simulink library "SUB_ECU_L4_MABX_HW_Interface_PIC_PB"  (R2018a)
settings: Solver=VariableStepAuto  StartTime=0.0  StopTime=10.0  RelTol=1e-3
PostLoadFcn:
  | , if any(exist('dsrtsu_mdlpostloadfcn', 'file') == [2, 3, 6]), try dsrtsu_mdlpostloadfcn('Execute', bdroot); catch fprintf('Error in PostLoadFcn (dsrtsu_mdlpostloadfcn) for model "%s":\n %s\n', bdroot, lasterr); end, end,
undefined symbols (not defined in the file or in its folder): CANR_PROPB_REAX_3_13_CHANNEL_APV, CANR_PROPB_REAX_4_13_CHANNEL_APV, CANR_PROPB_XPR_1_50_CHANNEL_APV, ENUM_CAN_RX_T, ENUM_CAN_TX_T, ENUM_REAX_OPERATION_MODE_T, ENUM_SIGNAL_HEALTH_T, ENUM_XBR_CONTROL_MODE_T, ENUM_XBR_EBI_MODE_T, ENUM_XBR_PASS_THROUGH_ACTIVE_T, ENUM_XBR_PRIORITY_T, ENUM_XPR_INHIBIT_PARK_MANUAL_T, ENUM_XPR_INHIBIT_UNPARK_MANUAL_T, ENUM_XPR_PARK_MANUAL_T, ENUM_XPR_UNPARK_MANUAL_T, PROPB_REAX_1_E4_DES_POS_SIG_SRC_APV, PROPB_REAX_1_E4_DESIRED_OPMODE_APV, PROPB_REAX_1_E4_DESIRED_POSITION_APV, PROPB_REAX_CHANNEL_APV, ptc_matlab_lib
libraries: PTC_MBDS_LIB x293, rtican x158, simulink x61, EmE_MBD_Blockset x38, rti1401lib_dio_type4 x14, simulink_need_slupdate x7, $bdroot x5, rti1401lib_adc_type4 x3, rtmapslib x3, dsa_tcpip_lib x2, SUB_ECU_L4_MABX_HW_Interface_PTC_1571 x1, rtitasklib x1
(part 29 of 49)

== system SUB_ECU_L4_MABX_HW_Interface_PIC_PB/INPUTS_PIC_PB/CAN_PIC_PB/CAN_RX_AIR1_31/RX_CAN_1 ==
  Enable : Inport
  AIR1 : rtican/RTICAN Receive (RX)   Reserved1=[]  Reserved2=[]  Reserved3=[]  Reserved4=[]  SfcnMessage=[]  Msg_Struct=[]  BoardTypeNo=[]  BoardNo=[]  ChannelNo=[]  Parameters=[]  DialogFcn=[]  UnitName=[]  Revision=[]  UnitValues=[]  DSProperties=struct('RTI',struct('Version',uint32(5),'BlockType',struct('isSLSource',uint8(1),'isSLSink',uint8(1),'isHWSource',uint8(0),'isHWSink',uint8(0),'isSetup',uint8(0),'isInline',uint8(1),'isNonInline',uint8(0),'isInterrupt',uint8(0),'isChannelwise',uint8(0)),'IOBoardType','RTICAN','UnitType','MESSAGE','Identifier','RX','DialogType','MSVC','BlockSet','RTICAN','SlaveProcessor','CAN'))  RTIBlockInterface=struct('OutputPortsWidth',int32([1 1 1 1 1 1 1 1 1 1 1]),'OutputPortsActive',ones(1,11),'OutputPortsName',{{'PneumaticSupplyPress','ParkingAnd_orTrailerAirPress','ServiceBrakeCircuit1AirPress','ServiceBrakeCircuit2AirPress','AuxEquipmentSupplyPress','AirSuspensionSupplyPress','AirCompressorStatus','PowertrainCircuitAirSupplyPress',['RX status'],['RX time'],['RX delta time']}},'OutputPortsDataType',{{'SS_DOUBLE','SS_DOUBLE','SS_DOUBLE','SS_DOUBLE','SS_DOUBLE','SS_DOUBLE','SS_DOUBLE','SS_DOUBLE','SS_DOUBLE','SS_DOUBLE','SS_DOUBLE'}},'OutputPortsLabel',{{'PneumaticSupplyPress','ParkingAnd_orTrailerAirPress','ServiceBrakeCircuit1AirPress','ServiceBrakeCircuit2AirPress','AuxEquipmentSupplyPress','AirSuspensionSupplyPress','AirCompressorStatus','PowertrainCircuitAirSupplyPress','','',''}},'OutputPortsLabelMode','ON','InputPortsWidth',int32(0),'InputPortsActive',0,'DialogFcn','rtican_message_interface_gui','BlockDisplay',{{'','center'}},'IconTransparency','on','ParameterTunableNames',{{}},'InitLevel',3,'BlockName',struct('Token',{{'AIR1'}}),'SampleTime',{{-1}},'TriggerPort',{{'none'}},'EnablePort',{{'yes'}})  RTIBlockParameters="struct('BoardTypeNo',{{1,'OFF',[]}},'BoardNo',{{1,'ON',[1 16]}},'ChannelNo',{{1,'ON',[1 2]}},'Parameters',{{struct('DataFileSupport',struct('DataFileSelectedMaster',1,'DataFileSelectedLocal',0,'DataFileName',['c:\\data\\truck1571\\dbc\\mabx_can1.dbc|c:\\data\\svn\\powertrainsys\\trunk\\src\\projects_rcp\\my2017_rcp\\dbc files\\j1939.dbc|'],'DataFileDate',{{{['24-Jan-2018 14:59:01']},{['24-Aug-2017 12:01:59']}}},'SelectedFile',['..\\svn\\powertrainsys\\trunk\\src\\projects_rcp\\my2017_rcp\\dbc files\\j1939.dbc']),'Options',struct('StatusSelected',1,'TimeSelected',1,'DeltaTimeSelected',1,'BytePortSelected',0,'MessageLengthSelected',0,'TriggerPort',struct('Selected',0,'TriggerType',0),'UserCoding',struct('Selected',0,'InterfaceFile','UserDecodingFile','FcnName','UserDecodeFcn','InportSelected',0,'InportWidth',1,'OutportSelected',0,'OutportWidth',1),'EnablePortSelected',1,'SignalOnPortnameSelected',1,'UseRXService',1),'Message',struct('MsgOnBlocknameSelected',1,'MsgName','AIR1','MsgIdFormat',1,'MsgId',419343921,'MsgLength',8,'NumSignals',8,'SampleTime',-1,'Signal',struct('SgnName',{'PneumaticSupplyPress','ParkingAnd_orTrailerAirPress','ServiceBrakeCircuit1AirPress','ServiceBrakeCircuit2AirPress','AuxEquipmentSupplyPress','AirSuspensionSupplyPress','AirCompressorStatus','PowertrainCircuitAirSupplyPress'},'SgnStartBit',{0,8,16,24,32,40,48,56},'SgnLength',{8,8,8,8,8,8,2,8},'SgnType',{0,0,0,0,0,0,0,0},'ModeValue',{-1,-1,-1,-1,-1,-1,-1,-1},'DataType',{0,0,0,0,0,0,0,0},'ByteLayout',{0,0,0,0,0,0,0,0},'Factor',{8,8,8,8,8,8,1,8},'Offset',{0,0,0,0,0,0,0,0},'SgnComment',{{['The pneumatic pressure in the main reservoir, sometimes referred to as the wet tank.']},{['The pneumatic pressure in the circuit or reservoir for the parking brake and/or the trailer supply.']},{['The pneumatic pressure in the primary service brake circuit or reservoir, supplying the rear axle.']},{['The pneumatic pressure in the secondary service brake circuit or reservoir, supplying the front axle.']},{['The pneumatic pressure in the auxiliary circuit.']},{['The pneumatic pressure in the circuit for the electronically controlled air suspension system.']},{['Indicates whether the air compressor is actively compressing air.  ' char(10) '' char(10) '00     Compressor not active' char(10) '01     Compressor active' char(10) '10     Error indicator' char(10) '11     Not available']},{['Supply pressure to carry the pressure information for the powertrain circuit. This circuit typically would feed powertrain components such as throttles, gearbox actuators and aftertreatment actuators for EGR and SCR systems.']}},'SgnUnit',{'kPa','kPa','kPa','kPa','kPa','kPa','','kPa'},'Min',{0,0,0,0,0,0,0,0},'Max',{2000,2000,2000,2000,2000,2000,3,2000},'SLDataType',{'SS_DOUBLE','SS_DOUBLE','SS_DOUBLE','SS_DOUBLE','SS_DOUBLE','SS_DOUBLE','SS_DOUBLE','SS_DOUBLE'}),'MsgIdNumFormat',1,'MsgComment',{{['Air Supply Pressure' char(10) 'Air Supply Pressure']}}),'Version',1.2,'general',struct('isFromLib',0)),'OFF',[]}},'GroupId',{{struct('Group',{{'RTICAN'}},'No',1,'Behavior',{{'NAMECHANGE'}},'BlockType',{{'SINK'}},'NameChangeFlag',0),'OFF',[]}},'SFcnRTICANMessage',{{struct('MsgType','RX','SFcnPortType','Scalar','MsgName','AIR1','MsgIdFormat','XTD','MsgId',419343921,'MsgLength',8,'NumSignals',8,'SampleTime',-1,'Signal',struct('SgnName',{'PneumaticSupplyPress','ParkingAnd_orTrailerAirPress','ServiceBrakeCircuit1AirPress','ServiceBrakeCircuit2AirPress','AuxEquipmentSupplyPress','AirSuspensionSupplyPress','AirCompressorStatus','PowertrainCircuitAirSupplyPress'},'SgnStartBit',{0,8,16,24,32,40,48,56},'SgnLength',{8,8,8,8,8,8,2,8},'SgnType',{'standard','standard','standard','standard','standard','standard','standard','standard'},'ModeValue',{-1,-1,-1,-1,-1,-1,-1,-1},'DataType',{['unsigned int'],['unsigned int'],['unsigned int'],['unsigned int'],['unsigned int'],['unsigned int'],['unsigned int'],['unsigned int']},'ByteLayout',{['little endian'],['little endian'],['little endian'],['little endian'],['little endian'],['little endian'],['little endian'],['little endian']},'Factor',{8,8,8,8,8,8,1,8},'Offset',{0,0,0,0,0,0,0,0},'SLDataType',{'SS_DOUBLE','SS_DOUBLE','SS_DOUBLE','SS_DOUBLE','SS_DOUBLE','SS_DOUBLE','SS_DOUBLE','SS_DOUBLE'}),'StatusSelected','yes','TimeSelected','yes','DeltaTimeSelected','yes','BytePortSelected','no','MessageLengthSelected','no','TriggerPort',struct('Selected','no','TriggerType',0),'UserCoding',struct('Selected','no','InterfaceFile','UserDecodingFile','FcnName','UserDecodeFcn','InportSelected','no','InportWidth',1,'OutportSelected','no','OutportWidth',1),'EnablePortSelected','yes','UseRXService','yes','BoardType','DS1','BoardNo',1,'ControllerNo',1),'OFF',[]}},'TLCFileName',{{'rtican_rx_message','OFF',[]}})"  RTISFcnParameters=struct('SFcnRTICANMessage','struct','TLCFileName','char')  RTIBlockParaDefault=struct('BoardTypeNo',4302,'BoardNo',1,'ChannelNo',1,'Parameters',struct('DataFileSupport',struct('DataFileSelectedMaster',0,'DataFileSelectedLocal',0,'DataFileName','','DataFileDate','','SelectedFile',['<no file selected>']),'Options',struct('StatusSelected',1,'TimeSelected',1,'DeltaTimeSelected',1,'BytePortSelected',0,'MessageLengthSelected',0,'TriggerPort',struct('Selected',0,'TriggerType','rising'),'UserCoding',struct('Selected',0,'InterfaceFile','UserDecodingFile','FcnName','UserDecodeFcn','InportSelected',0,'InportWidth',1,'OutportSelected',0,'OutportWidth',1),'EnablePortSelected',0,'SignalOnPortnameSelected',1,'UseRXService',0),'Message',struct('MsgOnBlocknameSelected',0,'MsgName',['RX Message'],'MsgIdFormat',0,'MsgId',100,'MsgLength',8,'NumSignals',1,'SampleTime',-1,'Signal',struct('SgnName',['RX signal'],'SgnStartBit',0,'SgnLength',8,'SgnType',0,'ModeValue',-1,'DataType',0,'SLDataType','SS_DOUBLE','ByteLayout',0,'Factor',1,'Offset',0,'Min',0,'Max',255,'SgnComment',{{}},'SgnUnit',''),'MsgIdNumFormat',0,'MsgComment',{{''}}),'Version',1.2,'general',struct('isFromLib',1)),'GroupId',struct('Group',{{'RTICAN'}},'No',1,'Behavior',{{'NAMECHANGE'}},'BlockType',{{'SINK'}},'NameChangeFlag',0),'SFcnRTICANMessage',struct('MsgType','RX','MsgName',['RX Message'],'MsgIdFormat','STD','MsgId',100,'MsgLength',8,'NumSignals',1,'SampleTime',-1,'Signal',struct('SgnName',['RX signal'],'SgnStartBit',0,'SgnLength',8,'SgnType','standard','ModeValue',-1,'DataType',['unsigned int'],'ByteLayout',['little endian'],'SLDataType','SS_DOUBLE','Factor',1,'Offset',0),'StatusSelected','yes','TimeSelected','yes','DeltaTimeSelected','yes','BytePortSelected','no','MessageLengthSelected','no','EnablePortSelected','no','UserCoding',struct('Selected','no','InterfaceFile','UserDecodingFile','FcnName','UserDecodeFcn','InportSelected','no','InportWidth',1,'OutportSelected','no','OutportWidth',1),'TriggerPort',struct('Selected','no','TriggerType','rising'),'UseRXService','no','BoardType','DS4302','BoardNo',1,'ControllerNo',1,'SFcnPortType','Scalar'),'TLCFileName','rtican_rx_message')
      settings: AttributesFormatString=Group Id: RTICAN1\n  SourceProductName=dSPACE RTI CAN Blockset
  Bus Creator : BusCreator  Inputs=8
  Bus Creator3 : BusCreator  Inputs=4
  Data Type Conversion10 : DataTypeConversion  OutDataTypeStr=double  SaturateOnIntegerOverflow=on
  Data Type Conversion8 : DataTypeConversion  OutDataTypeStr=boolean  SaturateOnIntegerOverflow=on
  Data Type Conversion9 : DataTypeConversion  OutDataTypeStr=double  SaturateOnIntegerOverflow=on
  AIR1_31 : Outport
  wires:
  Bus Creator3/1 -> AIR1_31/1  "AIR1_31"
  Bus Creator/1 -> Bus Creator3/1  "AIR1_31Data"
  Enable/1 -> AIR1/Enable
  AIR1/11 -> Data Type Conversion10/1
  AIR1/10 -> Data Type Conversion9/1
  AIR1/9 -> Data Type Conversion8/1
  Data Type Conversion8/1 -> Bus Creator3/2  "RX_status"
  Data Type Conversion10/1 -> Bus Creator3/4  "RX_delta_time"
  Data Type Conversion9/1 -> Bus Creator3/3  "RX_time"
  AIR1/1 -> Bus Creator/1  "PneumaticSupplyPress"
  AIR1/2 -> Bus Creator/2  "ParkingAnd_orTrailerAirPress"
  AIR1/3 -> Bus Creator/3  "ServiceBrakeCircuit1AirPress"
  AIR1/4 -> Bus Creator/4  "ServiceBrakeCircuit2AirPress"
  AIR1/5 -> Bus Creator/5  "AuxEquipmentSupplyPress"
  AIR1/6 -> Bus Creator/6  "AirSuspensionSupplyPress"
  AIR1/7 -> Bus Creator/7  "AirCompressorStatus"
  AIR1/8 -> Bus Creator/8  "PowertrainCircuitAirSupplyPress"

== system SUB_ECU_L4_MABX_HW_Interface_PIC_PB/INPUTS_PIC_PB/CAN_PIC_PB/CAN_RX_AMB_00/RX_CAN_1 ==
  Enable : Inport
  AMB : rtican/RTICAN Receive (RX)   Reserved1=[]  Reserved2=[]  Reserved3=[]  Reserved4=[]  SfcnMessage=[]  Msg_Struct=[]  BoardTypeNo=[]  BoardNo=[]  ChannelNo=[]  Parameters=[]  DialogFcn=[]  UnitName=[]  Revision=[]  UnitValues=[]  DSProperties=struct('RTI',struct('Version',uint32(5),'BlockType',struct('isSLSource',uint8(1),'isSLSink',uint8(1),'isHWSource',uint8(0),'isHWSink',uint8(0),'isSetup',uint8(0),'isInline',uint8(1),'isNonInline',uint8(0),'isInterrupt',uint8(0),'isChannelwise',uint8(0)),'IOBoardType','RTICAN','UnitType','MESSAGE','Identifier','RX','DialogType','MSVC','BlockSet','RTICAN','SlaveProcessor','CAN'))  RTIBlockInterface=struct('OutputPortsWidth',int32([1 1 1 1 1 1 1 1]),'OutputPortsActive',[1 1 1 1 1 1 1 1],'OutputPortsName',{{'BarometricPress','CabInteriorTemp','AmbientAirTemp','EngAirIntakeTemp','RoadSurfaceTemp',['RX status'],['RX time'],['RX delta time']}},'OutputPortsDataType',{{'SS_DOUBLE','SS_DOUBLE','SS_DOUBLE','SS_DOUBLE','SS_DOUBLE','SS_DOUBLE','SS_DOUBLE','SS_DOUBLE'}},'OutputPortsLabel',{{'BarometricPress','CabInteriorTemp','AmbientAirTemp','EngAirIntakeTemp','RoadSurfaceTemp','','',''}},'OutputPortsLabelMode','ON','InputPortsWidth',int32(0),'InputPortsActive',0,'DialogFcn','rtican_message_interface_gui','BlockDisplay',{{'','center'}},'IconTransparency','on','ParameterTunableNames',{{}},'InitLevel',3,'BlockName',struct('Token',{{'AMB'}}),'SampleTime',{{-1}},'TriggerPort',{{'none'}},'EnablePort',{{'yes'}})  RTIBlockParameters="struct('BoardTypeNo',{{1,'OFF',[]}},'BoardNo',{{1,'ON',[1 16]}},'ChannelNo',{{1,'ON',[1 2]}},'Parameters',{{struct('DataFileSupport',struct('DataFileSelectedMaster',1,'DataFileSelectedLocal',0,'DataFileName',['c:\\data\\truck1571\\dbc\\mabx_can1.dbc|c:\\data\\svn\\powertrainsys\\trunk\\src\\projects_rcp\\my2017_rcp\\dbc files\\j1939.dbc|'],'DataFileDate',{{{['24-Jan-2018 14:59:01']},{['24-Aug-2017 12:01:59']}}},'SelectedFile',['<no file selected>']),'Options',struct('StatusSelected',1,'TimeSelected',1,'DeltaTimeSelected',1,'BytePortSelected',0,'MessageLengthSelected',0,'TriggerPort',struct('Selected',0,'TriggerType',0),'UserCoding',struct('Selected',0,'InterfaceFile','UserDecodingFile','FcnName','UserDecodeFcn','InportSelected',0,'InportWidth',1,'OutportSelected',0,'OutportWidth',1),'EnablePortSelected',1,'SignalOnPortnameSelected',1,'UseRXService',1),'Message',struct('MsgOnBlocknameSelected',1,'MsgName','AMB','MsgIdFormat',1,'MsgId',419362048,'MsgLength',8,'NumSignals',5,'SampleTime',-1,'Signal',struct('SgnName',{'BarometricPress','CabInteriorTemp','AmbientAirTemp','EngAirIntakeTemp','RoadSurfaceTemp'},'SgnStartBit',{0,8,24,40,48},'SgnLength',{8,16,16,8,16},'SgnType',{0,0,0,0,0},'ModeValue',{-1,-1,-1,-1,-1},'DataType',{0,0,0,0,0},'ByteLayout',{0,0,0,0,0},'Factor',{2^-1,2^-5,2^-5,1,2^-5},'Offset',{0,-273,-273,-40,-273},'SgnComment',{{['Absolute air pressure of the atmosphere.']},{['Temperature of air inside the part of the vehicle that encloses the driver and vehicle operating controls.' char(10) '' char(10) 'Note: See also SPN 1691.  SPN 1662 is an additional diagnostic SPN associated with cab temperature.']},{['Temperature of air surrounding vehicle.']},{['Temperature of air entering vehicle air induction system.']},{['Indicated temperature of road surface over which vehicle is operating.']}},'SgnUnit',{'kPa','°C','°C','°C','°C'},'Min',{0,-273,-273,-40,-273},'Max',{125,1734.96875,1734.96875,210,1734.96875},'SLDataType',{'SS_DOUBLE','SS_DOUBLE','SS_DOUBLE','SS_DOUBLE','SS_DOUBLE'}),'MsgIdNumFormat',1,'MsgComment',{{['Ambient Conditions']}}),'Version',1.2,'general',struct('isFromLib',0)),'OFF',[]}},'GroupId',{{struct('Group',{{'RTICAN'}},'No',1,'Behavior',{{'NAMECHANGE'}},'BlockType',{{'SINK'}},'NameChangeFlag',0),'OFF',[]}},'SFcnRTICANMessage',{{struct('MsgType','RX','SFcnPortType','Scalar','MsgName','AMB','MsgIdFormat','XTD','MsgId',419362048,'MsgLength',8,'NumSignals',5,'SampleTime',-1,'Signal',struct('SgnName',{'BarometricPress','CabInteriorTemp','AmbientAirTemp','EngAirIntakeTemp','RoadSurfaceTemp'},'SgnStartBit',{0,8,24,40,48},'SgnLength',{8,16,16,8,16},'SgnType',{'standard','standard','standard','standard','standard'},'ModeValue',{-1,-1,-1,-1,-1},'DataType',{['unsigned int'],['unsigned int'],['unsigned int'],['unsigned int'],['unsigned int']},'ByteLayout',{['little endian'],['little endian'],['little endian'],['little endian'],['little endian']},'Factor',{2^-1,2^-5,2^-5,1,2^-5},'Offset',{0,-273,-273,-40,-273},'SLDataType',{'SS_DOUBLE','SS_DOUBLE','SS_DOUBLE','SS_DOUBLE','SS_DOUBLE'}),'StatusSelected','yes','TimeSelected','yes','DeltaTimeSelected','yes','BytePortSelected','no','MessageLengthSelected','no','TriggerPort',struct('Selected','no','TriggerType',0),'UserCoding',struct('Selected','no','InterfaceFile','UserDecodingFile','FcnName','UserDecodeFcn','InportSelected','no','InportWidth',1,'OutportSelected','no','OutportWidth',1),'EnablePortSelected','yes','UseRXService','yes','BoardType','DS1','BoardNo',1,'ControllerNo',1),'OFF',[]}},'TLCFileName',{{'rtican_rx_message','OFF',[]}})"  RTISFcnParameters=struct('SFcnRTICANMessage','struct','TLCFileName','char')  RTIBlockParaDefault=struct('BoardTypeNo',4302,'BoardNo',1,'ChannelNo',1,'Parameters',struct('DataFileSupport',struct('DataFileSelectedMaster',0,'DataFileSelectedLocal',0,'DataFileName','','DataFileDate','','SelectedFile',['<no file selected>']),'Options',struct('StatusSelected',1,'TimeSelected',1,'DeltaTimeSelected',1,'BytePortSelected',0,'MessageLengthSelected',0,'TriggerPort',struct('Selected',0,'TriggerType','rising'),'UserCoding',struct('Selected',0,'InterfaceFile','UserDecodingFile','FcnName','UserDecodeFcn','InportSelected',0,'InportWidth',1,'OutportSelected',0,'OutportWidth',1),'EnablePortSelected',0,'SignalOnPortnameSelected',1,'UseRXService',0),'Message',struct('MsgOnBlocknameSelected',0,'MsgName',['RX Message'],'MsgIdFormat',0,'MsgId',100,'MsgLength',8,'NumSignals',1,'SampleTime',-1,'Signal',struct('SgnName',['RX signal'],'SgnStartBit',0,'SgnLength',8,'SgnType',0,'ModeValue',-1,'DataType',0,'SLDataType','SS_DOUBLE','ByteLayout',0,'Factor',1,'Offset',0,'Min',0,'Max',255,'SgnComment',{{}},'SgnUnit',''),'MsgIdNumFormat',0,'MsgComment',{{''}}),'Version',1.2,'general',struct('isFromLib',1)),'GroupId',struct('Group',{{'RTICAN'}},'No',1,'Behavior',{{'NAMECHANGE'}},'BlockType',{{'SINK'}},'NameChangeFlag',0),'SFcnRTICANMessage',struct('MsgType','RX','MsgName',['RX Message'],'MsgIdFormat','STD','MsgId',100,'MsgLength',8,'NumSignals',1,'SampleTime',-1,'Signal',struct('SgnName',['RX signal'],'SgnStartBit',0,'SgnLength',8,'SgnType','standard','ModeValue',-1,'DataType',['unsigned int'],'ByteLayout',['little endian'],'SLDataType','SS_DOUBLE','Factor',1,'Offset',0),'StatusSelected','yes','TimeSelected','yes','DeltaTimeSelected','yes','BytePortSelected','no','MessageLengthSelected','no','EnablePortSelected','no','UserCoding',struct('Selected','no','InterfaceFile','UserDecodingFile','FcnName','UserDecodeFcn','InportSelected','no','InportWidth',1,'OutportSelected','no','OutportWidth',1),'TriggerPort',struct('Selected','no','TriggerType','rising'),'UseRXService','no','BoardType','DS4302','BoardNo',1,'ControllerNo',1,'SFcnPortType','Scalar'),'TLCFileName','rtican_rx_message')
      settings: AttributesFormatString=Group Id: RTICAN1\n  SourceProductName=dSPACE RTI CAN Blockset
  Bus Creator : BusCreator  Inputs=5
  Bus Creator3 : BusCreator  Inputs=4
  Data Type Conversion10 : DataTypeConversion  OutDataTypeStr=double  SaturateOnIntegerOverflow=on
  Data Type Conversion8 : DataTypeConversion  OutDataTypeStr=boolean  SaturateOnIntegerOverflow=on
  Data Type Conversion9 : DataTypeConversion  OutDataTypeStr=double  SaturateOnIntegerOverflow=on
  AMB_00 : Outport
  wires:
  Data Type Conversion9/1 -> Bus Creator3/3  "RX_time"
  Data Type Conversion10/1 -> Bus Creator3/4  "RX_delta_time"
  Data Type Conversion8/1 -> Bus Creator3/2  "RX_status"
  AMB/6 -> Data Type Conversion8/1
  AMB/7 -> Data Type Conversion9/1
  AMB/8 -> Data Type Conversion10/1
  Enable/1 -> AMB/Enable
  Bus Creator/1 -> Bus Creator3/1  "AMB_00Data"
  Bus Creator3/1 -> AMB_00/1  "AMB_00"
  AMB/1 -> Bus Creator/1  "BarometricPress"
  AMB/2 -> Bus Creator/2  "CabInteriorTemp"
  AMB/3 -> Bus Creator/3  "AmbientAirTemp"
  AMB/4 -> Bus Creator/4  "EngAirIntakeTemp"
  AMB/5 -> Bus Creator/5  "RoadSurfaceTemp"

== system SUB_ECU_L4_MABX_HW_Interface_PIC_PB/INPUTS_PIC_PB/CAN_PIC_PB/CAN_RX_B2_31/RX_CAN_4 ==
  Enable : Inport
  B2 : rtican/RTICAN Receive (RX)   Reserved1=[]  Reserved2=[]  Reserved3=[]  Reserved4=[]  SfcnMessage=[]  Msg_Struct=[]  BoardTypeNo=[]  BoardNo=[]  ChannelNo=[]  Parameters=[]  DialogFcn=[]  UnitName=[]  Revision=[]  UnitValues=[]  DSProperties=struct('RTI',struct('Version',uint32(5),'BlockType',struct('isSLSource',uint8(1),'isSLSink',uint8(1),'isHWSource',uint8(0),'isHWSink',uint8(0),'isSetup',uint8(0),'isInline',uint8(1),'isNonInline',uint8(0),'isInterrupt',uint8(0),'isChannelwise',uint8(0)),'IOBoardType','RTICAN','UnitType','MESSAGE','Identifier','RX','DialogType','MSVC','BlockSet','RTICAN','SlaveProcessor','CAN'))  RTIBlockInterface=struct('OutputPortsWidth',int32([1 1 1 1 1]),'OutputPortsActive',[1 1 1 1 1],'OutputPortsName',{{'BrakeAppPressDemanded','BrakeSwitch2',['RX status'],['RX time'],['RX delta time']}},'OutputPortsDataType',{{'SS_DOUBLE','SS_DOUBLE','SS_DOUBLE','SS_DOUBLE','SS_DOUBLE'}},'OutputPortsLabel',{{'BrakeAppPressDemanded','BrakeSwitch2','','',''}},'OutputPortsLabelMode','ON','InputPortsWidth',int32(0),'InputPortsActive',0,'DialogFcn','rtican_message_interface_gui','BlockDisplay',{{'','center'}},'IconTransparency','on','ParameterTunableNames',{{}},'InitLevel',3,'BlockName',struct('Token',{{'B2'}}),'SampleTime',{{-1}},'TriggerPort',{{'none'}},'EnablePort',{{'yes'}})  RTIBlockParameters=struct('BoardTypeNo',{{1,'OFF',[]}},'BoardNo',{{1,'ON',[1 16]}},'ChannelNo',{{1,'ON',[1 2]}},'Parameters',{{struct('DataFileSupport',struct('DataFileSelectedMaster',1,'DataFileSelectedLocal',0,'DataFileName',['c:\users\gavin.coelho\repos\l4 svn\branches\gennaro\project_l4\src\projectlibrary\dbc\mabx_can1.dbc|c:\users\gavin.coelho\repos\l4 svn\branches\gennaro\project_l4\src\projectlibrary\dbc\j1939_famosdbcwithfusion.dbc|'],'DataFileDate',{{{['30-Jan-2018 09:46:08']},{''}}},'SelectedFile',['<no file selected>']),'Options',struct('StatusSelected',1,'TimeSelected',1,'DeltaTimeSelected',1,'BytePortSelected',0,'MessageLengthSelected',0,'TriggerPort',struct('Selected',0,'TriggerType',0),'UserCoding',struct('Selected',0,'InterfaceFile','UserDecodingFile','FcnName','UserDecodeFcn','InportSelected',0,'InportWidth',1,'OutportSelected',0,'OutportWidth',1),'EnablePortSelected',1,'SignalOnPortnameSelected',1,'UseRXService',1),'Message',struct('MsgOnBlocknameSelected',1,'MsgName','B2','MsgIdFormat',1,'MsgId',418451505,'MsgLength',8,'NumSignals',2,'SampleTime',-1,'Signal',struct('SgnName',{'BrakeAppPressDemanded','BrakeSwitch2'},'SgnStartBit',{0,16},'SgnLength',{16,2},'SgnType',{0,0},'ModeValue',{-1,-1},'DataType',{0,0},'ByteLayout',{0,0},'Factor',{0.1,1},'Offset',{0,0},'SgnComment',{{['Gage pressure of compressed air or fluid in vehicle braking system measured at the brake chamber when brake shoe (or']},{['Switch signal which indicates that the driver operated brake foot pedal is being pressed.']}},'SgnUnit',{'kPa',''},'Min',{0,0},'Max',{6425.5,3},'SLDataType',{'SS_DOUBLE','SS_DOUBLE'}),'MsgIdNumFormat',1,'MsgComment',{{'Brakes'}}),'Version',1.2,'general',struct('isFromLib',0)),'OFF',[]}},'GroupId',{{struct('Group',{{'RTICAN'}},'No',1,'Behavior',{{'NAMECHANGE'}},'BlockType',{{'SINK'}},'NameChangeFlag',0),'OFF',[]}},'SFcnRTICANMessage',{{struct('MsgType','RX','SFcnPortType','Scalar','MsgName','B2','MsgIdFormat','XTD','MsgId',418451505,'MsgLength',8,'NumSignals',2,'SampleTime',-1,'Signal',struct('SgnName',{'BrakeAppPressDemanded','BrakeSwitch2'},'SgnStartBit',{0,16},'SgnLength',{16,2},'SgnType',{'standard','standard'},'ModeValue',{-1,-1},'DataType',{['unsigned int'],['unsigned int']},'ByteLayout',{['little endian'],['little endian']},'Factor',{0.1,1},'Offset',{0,0},'SLDataType',{'SS_DOUBLE','SS_DOUBLE'}),'StatusSelected','yes','TimeSelected','yes','DeltaTimeSelected','yes','BytePortSelected','no','MessageLengthSelected','no','TriggerPort',struct('Selected','no','TriggerType',0),'UserCoding',struct('Selected','no','InterfaceFile','UserDecodingFile','FcnName','UserDecodeFcn','InportSelected','no','InportWidth',1,'OutportSelected','no','OutportWidth',1),'EnablePortSelected','yes','UseRXService','yes','BoardType','DS1','BoardNo',1,'ControllerNo',1),'OFF',[]}},'TLCFileName',{{'rtican_rx_message','OFF',[]}})  RTISFcnParameters=struct('SFcnRTICANMessage','struct','TLCFileName','char')  RTIBlockParaDefault=struct('BoardTypeNo',4302,'BoardNo',1,'ChannelNo',1,'Parameters',struct('DataFileSupport',struct('DataFileSelectedMaster',0,'DataFileSelectedLocal',0,'DataFileName','','DataFileDate','','SelectedFile',['<no file selected>']),'Options',struct('StatusSelected',1,'TimeSelected',1,'DeltaTimeSelected',1,'BytePortSelected',0,'MessageLengthSelected',0,'TriggerPort',struct('Selected',0,'TriggerType','rising'),'UserCoding',struct('Selected',0,'InterfaceFile','UserDecodingFile','FcnName','UserDecodeFcn','InportSelected',0,'InportWidth',1,'OutportSelected',0,'OutportWidth',1),'EnablePortSelected',0,'SignalOnPortnameSelected',1,'UseRXService',0),'Message',struct('MsgOnBlocknameSelected',0,'MsgName',['RX Message'],'MsgIdFormat',0,'MsgId',100,'MsgLength',8,'NumSignals',1,'SampleTime',-1,'Signal',struct('SgnName',['RX signal'],'SgnStartBit',0,'SgnLength',8,'SgnType',0,'ModeValue',-1,'DataType',0,'SLDataType','SS_DOUBLE','ByteLayout',0,'Factor',1,'Offset',0,'Min',0,'Max',255,'SgnComment',{{}},'SgnUnit',''),'MsgIdNumFormat',0,'MsgComment',{{''}}),'Version',1.2,'general',struct('isFromLib',1)),'GroupId',struct('Group',{{'RTICAN'}},'No',1,'Behavior',{{'NAMECHANGE'}},'BlockType',{{'SINK'}},'NameChangeFlag',0),'SFcnRTICANMessage',struct('MsgType','RX','MsgName',['RX Message'],'MsgIdFormat','STD','MsgId',100,'MsgLength',8,'NumSignals',1,'SampleTime',-1,'Signal',struct('SgnName',['RX signal'],'SgnStartBit',0,'SgnLength',8,'SgnType','standard','ModeValue',-1,'DataType',['unsigned int'],'ByteLayout',['little endian'],'SLDataType','SS_DOUBLE','Factor',1,'Offset',0),'StatusSelected','yes','TimeSelected','yes','DeltaTimeSelected','yes','BytePortSelected','no','MessageLengthSelected','no','EnablePortSelected','no','UserCoding',struct('Selected','no','InterfaceFile','UserDecodingFile','FcnName','UserDecodeFcn','InportSelected','no','InportWidth',1,'OutportSelected','no','OutportWidth',1),'TriggerPort',struct('Selected','no','TriggerType','rising'),'UseRXService','no','BoardType','DS4302','BoardNo',1,'ControllerNo',1,'SFcnPortType','Scalar'),'TLCFileName','rtican_rx_message')
      settings: AttributesFormatString=Group Id: RTICAN1\n  SourceProductName=dSPACE RTI CAN Blockset
  Bus Creator3 : BusCreator  Inputs=5
  Data Type Conversion10 : DataTypeConversion  OutDataTypeStr=double  SaturateOnIntegerOverflow=on
  Data Type Conversion8 : DataTypeConversion  OutDataTypeStr=boolean  SaturateOnIntegerOverflow=on
  Data Type Conversion9 : DataTypeConversion  OutDataTypeStr=double  SaturateOnIntegerOverflow=on
  B2_31 : Outport
  wires:
  B2/2 -> Bus Creator3/2  "BrakeSwitch2"
  B2/1 -> Bus Creator3/1  "BrakeAppPressDemanded"
  Data Type Conversion9/1 -> Bus Creator3/4  "RX_time"
  Data Type Conversion10/1 -> Bus Creator3/5  "RX_delta_time"
  Data Type Conversion8/1 -> Bus Creator3/3  "RX_status"
  B2/3 -> Data Type Conversion8/1
  B2/4 -> Data Type Conversion9/1
  B2/5 -> Data Type Conversion10/1
  Enable/1 -> B2/Enable
  Bus Creator3/1 -> B2_31/1  "SystemTime_01"
